simulink model "Orangery"  (R2015a)
settings: configuration reference "GlobalConfig" (kept outside this file)
PreLoadFcn:
  | modelPreLoadClbck
InitFcn:
  | modelPreLoadClbck
undefined symbols (not defined in the file): Geom_GlassThick, Geom_RoofThick, Geom_Square_Glass_Roof, Geom_Square_Glass_Sides, Geom_Square_Roof, Geom_Square_Wall_Aboveground, Geom_Square_Wall_Underground, Geom_Volume, Geom_WallThick
libraries: fl_lib x30, nesl_utility x3
settings Model: CovSFcnEnable=off  Creator=Oleg_2  LastModifiedBy=Oleg
settings ConfigSetRef: SourceLocation=Base Workspace

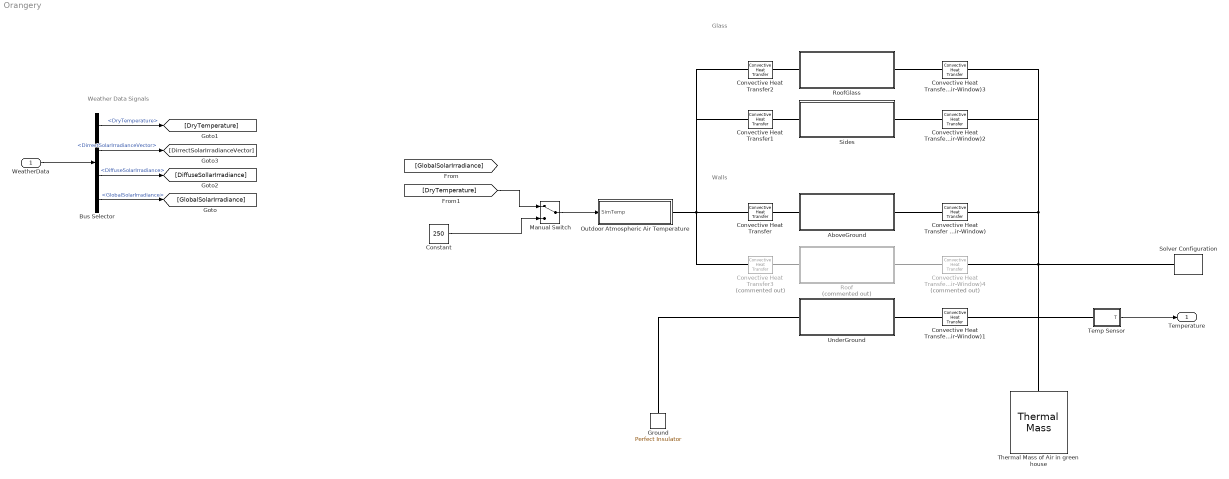
== system Orangery ==
  note: Glass
  note: Walls
  note: Weather Data Signals
  WeatherData : Inport  OutDataTypeStr=Bus: WeatherData
  AboveGround : Subsystem
  Bus Selector : BusSelector  OutputSignals=DryTemperature,DirrectSolarIrradianceVector,DiffuseSolarIrradiance,GlobalSolarIrradiance
  Constant : Constant  Value=250
  Convective Heat Transfer : fl_lib/Thermal/Thermal Elements/Convective Heat Transfer  area=Geom_Square_Wall_Underground m^2  heat_tr_coeff=32 W/(m^2 * K)  Q_specify=off  Q_priority=High  Q=0 J/s  T_specify=off  T_priority=High  T=0 K
      settings: AttributesFormatString=|
      | Heat_tr_coeff: %<heat_tr_coeff>
      | Area: %<area>
  Convective Heat Transfer (Air-Window) : fl_lib/Thermal/Thermal Elements/Convective Heat Transfer  area=Geom_Square_Wall_Aboveground m^2  heat_tr_coeff=15 W/(m^2 * K)  Q_specify=off  Q_priority=High  Q=0 J/s  T_specify=off  T_priority=High  T=0 K
      settings: AttributesFormatString=|
      | Heat_tr_coeff: %<heat_tr_coeff>
      | Area: %<area>
  Convective Heat Transfer (Air-Window)1 : fl_lib/Thermal/Thermal Elements/Convective Heat Transfer  area=Geom_Square_Wall_Underground m^2  heat_tr_coeff=15 W/(m^2 * K)  Q_specify=off  Q_priority=High  Q=0 J/s  T_specify=off  T_priority=High  T=0 K
      settings: AttributesFormatString=|
      | Heat_tr_coeff: %<heat_tr_coeff>
      | Area: %<area>
  Convective Heat Transfer (Air-Window)2 : fl_lib/Thermal/Thermal Elements/Convective Heat Transfer  area=Geom_Square_Glass_Sides m^2  heat_tr_coeff=15 W/(m^2 * K)  Q_specify=off  Q_priority=High  Q=0 J/s  T_specify=off  T_priority=High  T=0 K
      settings: AttributesFormatString=|
      | Heat_tr_coeff: %<heat_tr_coeff>
      | Area: %<area>
  Convective Heat Transfer (Air-Window)3 : fl_lib/Thermal/Thermal Elements/Convective Heat Transfer  area=Geom_Square_Glass_Roof m^2  heat_tr_coeff=15 W/(m^2 * K)  Q_specify=off  Q_priority=High  Q=0 J/s  T_specify=off  T_priority=High  T=0 K
      settings: AttributesFormatString=|
      | Heat_tr_coeff: %<heat_tr_coeff>
      | Area: %<area>
  Convective Heat Transfer (Air-Window)4 : fl_lib/Thermal/Thermal Elements/Convective Heat Transfer  Commented=on  area=Geom_Square_Roof m^2  heat_tr_coeff=15 W/(m^2 * K)  Q_specify=off  Q_priority=High  Q=0 J/s  T_specify=off  T_priority=High  T=0 K
      settings: AttributesFormatString=|
      | Heat_tr_coeff: %<heat_tr_coeff>
      | Area: %<area>
  Convective Heat Transfer1 : fl_lib/Thermal/Thermal Elements/Convective Heat Transfer  area=Geom_Square_Glass_Sides m^2  heat_tr_coeff=32 W/(m^2 * K)  Q_specify=off  Q_priority=High  Q=0 J/s  T_specify=off  T_priority=High  T=0 K
      settings: AttributesFormatString=|
      | Heat_tr_coeff: %<heat_tr_coeff>
      | Area: %<area>
  Convective Heat Transfer2 : fl_lib/Thermal/Thermal Elements/Convective Heat Transfer  area=Geom_Square_Glass_Roof m^2  heat_tr_coeff=32 W/(m^2 * K)  Q_specify=off  Q_priority=High  Q=0 J/s  T_specify=off  T_priority=High  T=0 K
      settings: AttributesFormatString=|
      | Heat_tr_coeff: %<heat_tr_coeff>
      | Area: %<area>
  Convective Heat Transfer3 : fl_lib/Thermal/Thermal Elements/Convective Heat Transfer  Commented=on  area=Geom_Square_Roof m^2  heat_tr_coeff=32 W/(m^2 * K)  Q_specify=off  Q_priority=High  Q=0 J/s  T_specify=off  T_priority=High  T=0 K
      settings: AttributesFormatString=|
      | Heat_tr_coeff: %<heat_tr_coeff>
      | Area: %<area>
  Ground : fl_lib/Thermal/Thermal Elements/Perfect Insulator  T_specify=off  T_priority=High  T=0 K
  Manual Switch : ManualSwitch
  Outdoor Atmospheric Air Temperature : Subsystem
  Roof : Subsystem  Commented=on
  RoofGlass : Subsystem
  Sides : Subsystem
  Solver Configuration : nesl_utility/Solver Configuration  PhysicalDomain=network_engine_domain  SubClassName=solver  LeftPortType=input  RightPortType=generic  Accelerate=off  Tones=[]  Harmonics=[]  SimulateNoise=off  Profile=off  UseLocalSampling=off  EnableSwitchedLinearOptims=on  FrequencyDomain=off  UseCCode=off  RelTol=0.001  AbsTol=1e-06  MinStep=1e-09  ToWorkspace=off  RevertToSquareIcSolve=off  NumHomotopyIterations=100  DoDC=on  ResidualTolerance=1e-16  UseLocalSolver=on  LocalSolverChoice=NE_TRAPEZOIDAL_ADVANCER  LocalSolverSampleTime=60  DoFixedCost=on  MaxNonlinIter=10  MaxModeIter=2  LinearAlgebra=Sparse  DelaysMemoryBudget=1024  AutomaticFiltering=on  FilteringTimeConstant=0.001
  Temp Sensor : Subsystem
  Thermal Mass of Air in green house : fl_lib/Thermal/Thermal Elements/Thermal Mass  mass=Geom_Volume * 1.293 kg  sp_heat=1006 J/kg/K  Q_specify=on  Q_priority=High  Q=0 J/s  T_specify=on  T_priority=High  T=273+15 K
  UnderGround : Subsystem
  Temperature : Outport
  wires:
  WeatherData/1 -> Bus Selector/1
  Bus Selector/4 -> [GlobalSolarIrradiance]  "<GlobalSolarIrradiance>"
  Bus Selector/1 -> [DryTemperature]  "<DryTemperature>"
  Bus Selector/2 -> [DirrectSolarIrradianceVector]  "<DirrectSolarIrradianceVector>"
  Bus Selector/3 -> [DiffuseSollarIrradiance]  "<DiffuseSolarIrradiance>"
  [DryTemperature] -> Manual Switch/1
  Constant/1 -> Manual Switch/2
  Temp Sensor/1(T) -> Temperature/1
  Manual Switch/1 -> Outdoor Atmospheric Air Temperature/1(SimTemp)
  connections:
  Solver Configuration/RConn1 -- Thermal Mass of Air in green house/LConn1 -- Temp Sensor/LConn1 -- Convective Heat Transfer (Air-Window)1/RConn1 -- Convective Heat Transfer (Air-Window)/RConn1 -- Convective Heat Transfer (Air-Window)2/RConn1 -- Convective Heat Transfer (Air-Window)3/RConn1 -- Convective Heat Transfer (Air-Window)4/RConn1
  Convective Heat Transfer/LConn1 -- Convective Heat Transfer3/LConn1 -- Outdoor Atmospheric Air Temperature/RConn1 -- Convective Heat Transfer2/LConn1 -- Convective Heat Transfer1/LConn1
  Convective Heat Transfer/RConn1 -- AboveGround/LConn1
  AboveGround/RConn1 -- Convective Heat Transfer (Air-Window)/LConn1
  Ground/LConn1 -- UnderGround/LConn1
  UnderGround/RConn1 -- Convective Heat Transfer (Air-Window)1/LConn1
  Convective Heat Transfer (Air-Window)2/LConn1 -- Sides/RConn1
  Convective Heat Transfer1/RConn1 -- Sides/LConn1
  Convective Heat Transfer2/RConn1 -- RoofGlass/LConn1
  Convective Heat Transfer (Air-Window)3/LConn1 -- RoofGlass/RConn1
  Convective Heat Transfer3/RConn1 -- Roof/LConn1
  Roof/RConn1 -- Convective Heat Transfer (Air-Window)4/LConn1

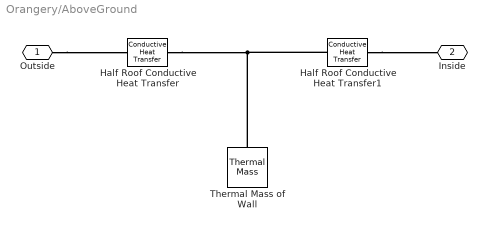
== system Orangery/AboveGround ==
  Half Roof Conductive Heat Transfer : fl_lib/Thermal/Thermal Elements/Conductive Heat Transfer  area=Geom_Square_Wall_Aboveground m^2  thickness=Geom_WallThick/2 m  th_cond=0.05 W/(m*K)  Q_specify=off  Q_priority=High  Q=0 J/s  T_specify=off  T_priority=High  T=0 K
      settings: AttributesFormatString=|
      | Therm Conduction: %<th_cond>
      | Area: %<area>
      | Thick: %<thickness>
  Half Roof Conductive Heat Transfer1 : fl_lib/Thermal/Thermal Elements/Conductive Heat Transfer  area=Geom_Square_Wall_Aboveground m^2  thickness=Geom_WallThick/2 m  th_cond=0.05 W/(m*K)  Q_specify=off  Q_priority=High  Q=0 J/s  T_specify=off  T_priority=High  T=0 K
      settings: AttributesFormatString=|
      | Therm Conduction: %<th_cond>
      | Area: %<area>
      | Thick: %<thickness>
  Thermal Mass of Wall : fl_lib/Thermal/Thermal Elements/Thermal Mass  mass=Geom_Square_Wall_Aboveground * Geom_WallThick*1000 kg  sp_heat=920 J/kg/K  Q_specify=off  Q_priority=High  Q=0 J/s  T_specify=on  T_priority=High  T=300 K
      settings: AttributesFormatString=|
      | Mass: %<mass>
      | Heat: %<sp_heat>
  Outside : PMIOPort  Port=1  Side=Left
  Inside : PMIOPort  Port=2  Side=Right
  connections:
  Half Roof Conductive Heat Transfer1/RConn1 -- Inside/RConn1
  Outside/RConn1 -- Half Roof Conductive Heat Transfer/LConn1
  Half Roof Conductive Heat Transfer/RConn1 -- Half Roof Conductive Heat Transfer1/LConn1 -- Thermal Mass of Wall/LConn1

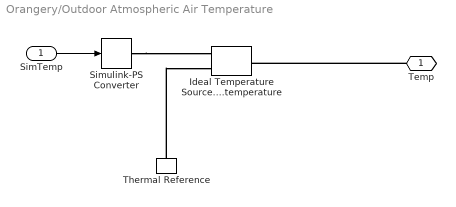
== system Orangery/Outdoor Atmospheric Air Temperature ==
  SimTemp : Inport
  Ideal Temperature Source. Outdoor temperature : fl_lib/Thermal/Thermal Sources/Ideal Temperature Source
  Simulink-PS Converter : nesl_utility/Simulink-PS Converter  PhysicalDomain=network_engine_domain  SubClassName=ps_input  LeftPortType=input  RightPortType=output  PseudoPeriodic=off  Frequencies=[]  NoiseDistribution=none  NoiseParameters=[]  Unit=K  AffineConversion=on  InputFiltering=off  SimscapeFilterOrder=1  InputFilterTimeConstant=.001  UdotUserProvided=1
  Thermal Reference : fl_lib/Thermal/Thermal Elements/Thermal Reference
  Temp : PMIOPort  Port=1  Side=Right
  wires:
  SimTemp/1 -> Simulink-PS Converter/1
  connections:
  Simulink-PS Converter/RConn1 -- Ideal Temperature Source. Outdoor temperature/RConn1
  Thermal Reference/LConn1 -- Ideal Temperature Source. Outdoor temperature/RConn2
  Temp/RConn1 -- Ideal Temperature Source. Outdoor temperature/LConn1

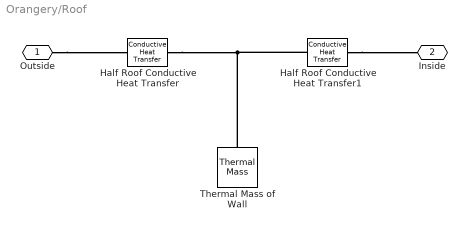
== system Orangery/Roof ==
  Half Roof Conductive Heat Transfer : fl_lib/Thermal/Thermal Elements/Conductive Heat Transfer  area=Geom_Square_Roof m^2  thickness=Geom_WallThick/2 m  th_cond=0.5 W/(m*K)  Q_specify=off  Q_priority=High  Q=0 J/s  T_specify=off  T_priority=High  T=0 K
      settings: AttributesFormatString=|
      | Therm Conduction: %<th_cond>
      | Area: %<area>
      | Thick: %<thickness>
  Half Roof Conductive Heat Transfer1 : fl_lib/Thermal/Thermal Elements/Conductive Heat Transfer  area=Geom_Square_Roof m^2  thickness=Geom_WallThick/2 m  th_cond=0.5 W/(m*K)  Q_specify=off  Q_priority=High  Q=0 J/s  T_specify=off  T_priority=High  T=0 K
      settings: AttributesFormatString=|
      | Therm Conduction: %<th_cond>
      | Area: %<area>
      | Thick: %<thickness>
  Thermal Mass of Wall : fl_lib/Thermal/Thermal Elements/Thermal Mass  mass=Geom_Square_Roof * Geom_RoofThick*10 kg  sp_heat=920 J/kg/K  Q_specify=off  Q_priority=High  Q=0 J/s  T_specify=on  T_priority=High  T=0 C
      settings: AttributesFormatString=|
      | Mass: %<mass>
      | Heat: %<sp_heat>
  Outside : PMIOPort  Port=1  Side=Left
  Inside : PMIOPort  Port=2  Side=Right
  connections:
  Half Roof Conductive Heat Transfer1/RConn1 -- Inside/RConn1
  Outside/RConn1 -- Half Roof Conductive Heat Transfer/LConn1
  Half Roof Conductive Heat Transfer/RConn1 -- Half Roof Conductive Heat Transfer1/LConn1 -- Thermal Mass of Wall/LConn1

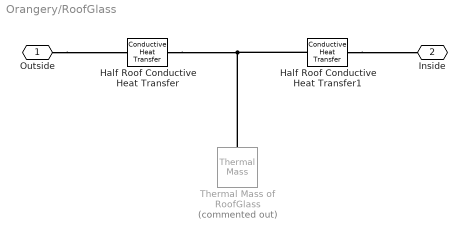
== system Orangery/RoofGlass ==
  Half Roof Conductive Heat Transfer : fl_lib/Thermal/Thermal Elements/Conductive Heat Transfer  area=Geom_Square_Glass_Roof m^2  thickness=Geom_GlassThick/2 m  th_cond=1 W/(m*K)  Q_specify=off  Q_priority=High  Q=0 J/s  T_specify=off  T_priority=High  T=0 K
      settings: AttributesFormatString=|
      | Therm Conduction: %<th_cond>
      | Area: %<area>
      | Thick: %<thickness>
  Half Roof Conductive Heat Transfer1 : fl_lib/Thermal/Thermal Elements/Conductive Heat Transfer  area=Geom_Square_Glass_Roof m^2  thickness=Geom_GlassThick/2 m  th_cond=1 W/(m*K)  Q_specify=off  Q_priority=High  Q=0 J/s  T_specify=off  T_priority=High  T=0 K
      settings: AttributesFormatString=|
      | Therm Conduction: %<th_cond>
      | Area: %<area>
      | Thick: %<thickness>
  Thermal Mass of RoofGlass : fl_lib/Thermal/Thermal Elements/Thermal Mass  Commented=on  mass=Geom_Square_Glass_Roof * Geom_GlassThick kg  sp_heat=920 J/kg/K  Q_specify=off  Q_priority=High  Q=0 J/s  T_specify=on  T_priority=High  T=0 C
      settings: AttributesFormatString=|
      | Mass: %<mass>
      | Heat: %<sp_heat>
  Outside : PMIOPort  Port=1  Side=Left
  Inside : PMIOPort  Port=2  Side=Right
  connections:
  Half Roof Conductive Heat Transfer1/RConn1 -- Inside/RConn1
  Outside/RConn1 -- Half Roof Conductive Heat Transfer/LConn1
  Half Roof Conductive Heat Transfer/RConn1 -- Half Roof Conductive Heat Transfer1/LConn1 -- Thermal Mass of RoofGlass/LConn1

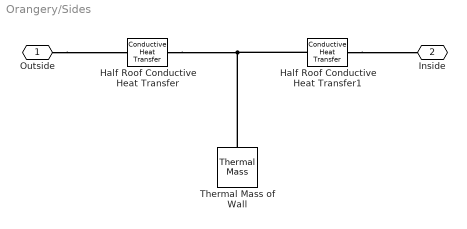
== system Orangery/Sides ==
  Half Roof Conductive Heat Transfer : fl_lib/Thermal/Thermal Elements/Conductive Heat Transfer  area=Geom_Square_Glass_Sides m^2  thickness=Geom_GlassThick/2 m  th_cond=1 W/(m*K)  Q_specify=off  Q_priority=High  Q=0 J/s  T_specify=off  T_priority=High  T=0 K
      settings: AttributesFormatString=|
      | Therm Conduction: %<th_cond>
      | Area: %<area>
      | Thick: %<thickness>
  Half Roof Conductive Heat Transfer1 : fl_lib/Thermal/Thermal Elements/Conductive Heat Transfer  area=Geom_Square_Glass_Sides m^2  thickness=Geom_GlassThick/2 m  th_cond=1 W/(m*K)  Q_specify=off  Q_priority=High  Q=0 J/s  T_specify=off  T_priority=High  T=0 K
      settings: AttributesFormatString=|
      | Therm Conduction: %<th_cond>
      | Area: %<area>
      | Thick: %<thickness>
  Thermal Mass of Wall : fl_lib/Thermal/Thermal Elements/Thermal Mass  mass=Geom_Square_Glass_Sides * Geom_GlassThick*1 kg  sp_heat=920 J/kg/K  Q_specify=off  Q_priority=High  Q=0 J/s  T_specify=on  T_priority=High  T=273 K
      settings: AttributesFormatString=|
      | Mass: %<mass>
      | Heat: %<sp_heat>
  Outside : PMIOPort  Port=1  Side=Left
  Inside : PMIOPort  Port=2  Side=Right
  connections:
  Half Roof Conductive Heat Transfer1/RConn1 -- Inside/RConn1
  Outside/RConn1 -- Half Roof Conductive Heat Transfer/LConn1
  Half Roof Conductive Heat Transfer/RConn1 -- Half Roof Conductive Heat Transfer1/LConn1 -- Thermal Mass of Wall/LConn1

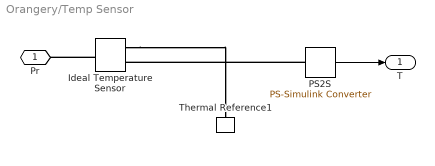
== system Orangery/Temp Sensor ==
  Ideal Temperature Sensor : fl_lib/Thermal/Thermal Sensors/Ideal Temperature Sensor
  PS2S : nesl_utility/PS-Simulink Converter  PhysicalDomain=network_engine_domain  SubClassName=ps_output  LeftPortType=input  RightPortType=output  PseudoPeriodic=off  Frequencies=[]  Unit=K  AffineConversion=off
  Thermal Reference1 : fl_lib/Thermal/Thermal Elements/Thermal Reference
  Pr : PMIOPort  Port=1  Side=Left
  T : Outport
  wires:
  PS2S/1 -> T/1
  connections:
  Ideal Temperature Sensor/RConn1 -- Thermal Reference1/LConn1
  Ideal Temperature Sensor/LConn1 -- Pr/RConn1
  PS2S/LConn1 -- Ideal Temperature Sensor/RConn2

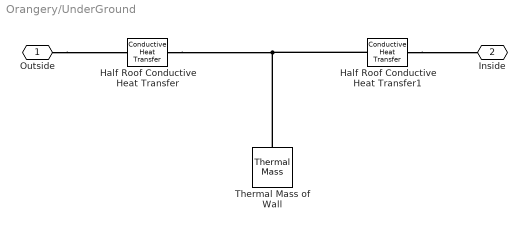
== system Orangery/UnderGround ==
  Half Roof Conductive Heat Transfer : fl_lib/Thermal/Thermal Elements/Conductive Heat Transfer  area=Geom_Square_Wall_Underground m^2  thickness=Geom_WallThick/2 m  th_cond=0.6 W/(m*K)  Q_specify=off  Q_priority=High  Q=0 J/s  T_specify=off  T_priority=High  T=0 K
      settings: AttributesFormatString=|
      | Therm Conduction: %<th_cond>
      | Area: %<area>
      | Thick: %<thickness>
  Half Roof Conductive Heat Transfer1 : fl_lib/Thermal/Thermal Elements/Conductive Heat Transfer  area=Geom_Square_Wall_Underground m^2  thickness=Geom_WallThick/2 m  th_cond=0.6 W/(m*K)  Q_specify=off  Q_priority=High  Q=0 J/s  T_specify=off  T_priority=High  T=0 K
      settings: AttributesFormatString=|
      | Therm Conduction: %<th_cond>
      | Area: %<area>
      | Thick: %<thickness>
  Thermal Mass of Wall : fl_lib/Thermal/Thermal Elements/Thermal Mass  mass=Geom_Square_Wall_Underground * Geom_WallThick*1000 kg  sp_heat=920 J/kg/K  Q_specify=off  Q_priority=High  Q=0 J/s  T_specify=on  T_priority=High  T=273 K
      settings: AttributesFormatString=|
      | Mass: %<mass>
      | Heat: %<sp_heat>
  Outside : PMIOPort  Port=1  Side=Left
  Inside : PMIOPort  Port=2  Side=Right
  connections:
  Half Roof Conductive Heat Transfer1/RConn1 -- Inside/RConn1
  Outside/RConn1 -- Half Roof Conductive Heat Transfer/LConn1
  Half Roof Conductive Heat Transfer/RConn1 -- Thermal Mass of Wall/LConn1 -- Half Roof Conductive Heat Transfer1/LConn1
